simulink model "crane_sim"  (Simulink 8.3)
settings: Solver=ode45  StartTime=0.0  StopTime=100  RelTol=1e-3
undefined symbols (not defined in the file or in its folder): crane_ctrl, drawGantryCrane, P
settings Model: Creator=beard  LastModifiedBy=jhl48
settings OptimizationCC: ExpressionDepthLimit=2147483647  InitFltsAndDblsToZero=on
settings DebuggingCC: FcnCallInpInsideContextMsg=UseLocalSettings

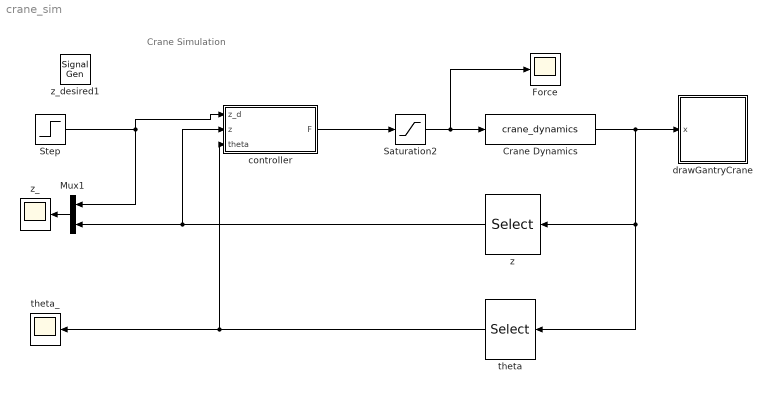
== system crane_sim ==
  note: Crane Simulation
  Crane Dynamics : S-Function  FunctionName=crane_dynamics  Parameters=P  EnableBusSupport=off
  Force : Scope
      settings: TimeRange=100  YMin=-1000  YMax=1250
  Mux1 : Mux  Inputs=2
  Saturation2 : Saturate  UpperLimit=P.F_max  LowerLimit=-P.F_max
  Step : Step  Time=20  After=7  SampleTime=0
  controller : Subsystem
  drawGantryCrane : Subsystem
      mask init:
      | bar = 20;
      | crane = [5 3];
      | L1 = 10;
      | R1 = 1;
      mask Display: image(imread('tv.jpg'))
  theta : Selector  InputPortWidth=4  Indices=[4]
  theta_ : Scope
      settings: TimeRange=100  YMin=-0.2  YMax=0.2
  z : Selector  InputPortWidth=4  Indices=[3]
  z_ : Scope
      settings: TimeRange=100  YMin=7  YMax=7  SaveName=ScopeData2
  z_desired1 : SignalGenerator  WaveForm=square  Amplitude=7  Frequency=.02
  wires:
  Crane Dynamics/1 -> theta/1, z/1, drawGantryCrane/1(x)
  controller/1(F) -> Saturation2/1
  Mux1/1 -> z_/1
  Saturation2/1 -> Crane Dynamics/1, Force/1
  Step/1 -> controller/1(z_d), Mux1/1
  z/1 -> controller/2(z), Mux1/2
  theta/1 -> controller/3(theta), theta_/1

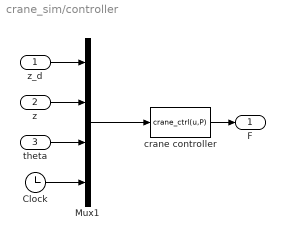
== system crane_sim/controller ==
  z_d : Inport
  z : Inport  Port=2
  theta : Inport  Port=3
  Clock : Clock
  Mux1 : Mux
  crane controller : MATLABFcn  MATLABFcn=crane_ctrl(u,P)  OutputDimensions=1  SampleTime=P.Ts
  F : Outport
  wires:
  crane controller/1 -> F/1
  z/1 -> Mux1/2
  z_d/1 -> Mux1/1
  Mux1/1 -> crane controller/1
  Clock/1 -> Mux1/4
  theta/1 -> Mux1/3

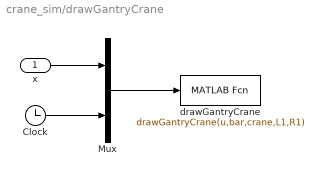
== system crane_sim/drawGantryCrane ==
  x : Inport
  Clock : Clock
  Mux : Mux  Inputs=2
  drawGantryCrane : MATLABFcn  MATLABFcn=drawGantryCrane(u,bar,crane,L1,R1)  OutputDimensions=0  SampleTime=0.1
  wires:
  Mux/1 -> drawGantryCrane/1
  x/1 -> Mux/1
  Clock/1 -> Mux/2
